simulink model "countersdemo"  (Simulink 6.0)
settings: Solver=FixedStepDiscrete  StartTime=0.0  StopTime=2  FixedStep=.01  RelTol=1e-3  AbsTol=1e-6
settings Model: Creator=The MathWorks Inc.  LastModifiedBy=batserve  ExtModeTrigMode=oneshot  ExtModeArmWhenConnect=off  ExtModeAutoUpdateStatusClock=off
settings DataIOCC: LimitDataPoints=off
settings OptimizationCC: BlockReduction=off  BooleanDataType=off
settings DebuggingCC: CheckExecutionContextPreStartOutputMsg=on  CheckExecutionContextRuntimeOutputMsg=on  SolverPrmCheckMsg=none
settings HardwareCC: TargetUnknown=on
settings RTWCC: SystemTargetFile=rt_ada_sim.tlc  MakeCommand=make_rtw -ada  TemplateMakefile=gnat_sim.tmf  ProcessScript=rt_ada_sim_make_rtw_hook
settings STFCustomTargetCC: TargetFcnLib=ansi_tfl_tmw.mat  GenFloatMathFcnCalls=ANSI_C  ModelReferenceCompliant=off  MatFileLogging=on  SystemTargetFile=rt_ada_sim.tlc

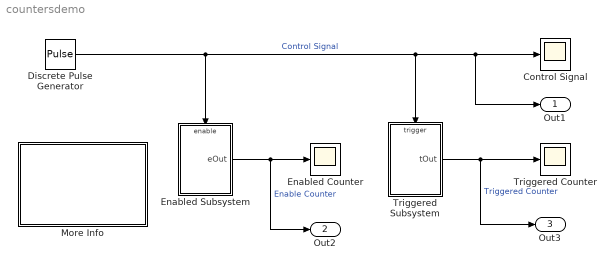
== system countersdemo ==
  Control Signal : Scope
      settings: YMin=-0.1  YMax=1.1  SaveName=Control_Signal  DataFormat=Array
  Discrete Pulse Generator : DiscretePulseGenerator  Period=40  PulseWidth=20  SampleTime=0.01
  Enabled Counter : Scope
      settings: TimeRange=2  YMin=-0.1  YMax=20  SaveName=Enabled_Counter  DataFormat=Array
  Enabled Subsystem : Subsystem  TreatAsAtomicUnit=on  PropExecContextAcrossSSBoundary=on
  More Info : Subsystem  PropExecContextAcrossSSBoundary=on
      mask Display: disp('Double click\nhere for\ninformation on\nthis demonstration')
  Triggered Counter : Scope
      settings: TimeRange=2  YMin=-0.1  YMax=4.1  SaveName=Triggered_Counter  DataFormat=Array
  Triggered Subsystem : Subsystem  TreatAsAtomicUnit=on  PropExecContextAcrossSSBoundary=on
  Out1 : Outport
  Out2 : Outport  Port=2
  Out3 : Outport  Port=3
  wires:
  Discrete Pulse Generator/1 -> Enabled Subsystem/Enable, Triggered Subsystem/Trigger, Control Signal/1, Out1/1  "Control Signal"
  Triggered Subsystem/1(tOut) -> Triggered Counter/1, Out3/1  "Triggered Counter"
  Enabled Subsystem/1(eOut) -> Enabled Counter/1, Out2/1  "Enable Counter"

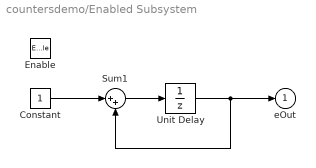
== system countersdemo/Enabled Subsystem ==
  Enable : EnablePort  StatesWhenEnabling=reset
  Constant : Constant
  Sum1 : Sum  Inputs=|++  SaturateOnIntegerOverflow=on  InputSameDT=on
  Unit Delay : UnitDelay  SampleTime=.01
  eOut : Outport  InitialOutput=0
  wires:
  Sum1/1 -> Unit Delay/1
  Constant/1 -> Sum1/1
  Unit Delay/1 -> eOut/1, Sum1/2

== system countersdemo/More Info ==
  note: Enabled Subsystem Demonstration
  note: This demonstration uses counter circuits to contrast the execution of
      | blocks in enabled subsystems and triggered subsystems for the same
      | control signal.  After running the simulation, the scope shows three plots.
      |
      | The first of these plots shows the control signal which is the output of the
      | discrete pulse generator.
      |
      | The second plot shows the output of the counter circuit in the enabled
      | subsystem.  The counter increments while the subsystem is enabled and
      | then holds its output when the subsystem is disabled.  The counter resets to
      | zero when the subsystem is re-enabled because the enable port was
      | configured to reset states when enabling.
      |
      | The third plot shows the output of the counter circuit in the triggered
      | subsystem.  The counter increments every rising edge of the control
      | signal.

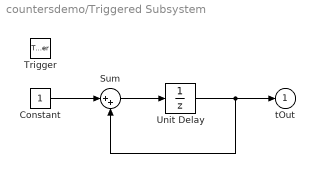
== system countersdemo/Triggered Subsystem ==
  Trigger : TriggerPort
  Constant : Constant
  Sum : Sum  Inputs=|++  SaturateOnIntegerOverflow=on  InputSameDT=on
  Unit Delay : UnitDelay  SampleTime=-1
  tOut : Outport  OutputWhenDisabled=reset  InitialOutput=0
  wires:
  Sum/1 -> Unit Delay/1
  Constant/1 -> Sum/1
  Unit Delay/1 -> tOut/1, Sum/2
